simulink model "CM660A_HwTq1Meas"  (R2013b)
settings: Solver=FixedStepDiscrete  StartTime=0.0  StopTime=20  FixedStep=0.002  RelTol=1e-3
undefined symbols (not defined in the file): ELECGLBPRM_HWTQOFFS_HWNWTMTR_F32, ELECGLBPRM_HWTQSATNLOWRLIM_HWNWTMTR_F32, ELECGLBPRM_HWTQSATNUPPRLIM_HWNWTMTR_F32, ELECGLBPRM_HWTQSCA_ULS_F32, ELECGLBPRM_NOFLT_CNT_U08, ELECGLBPRM_OFFSTRIMNOTPRFM_CNT_U08, ELECGLBPRM_PRTCLFLT_CNT_U08, ELECGLBPRM_SNSRINTFLT_CNT_U08, HwTq1MeasHwTq1PrtclFltFailStep, HwTq1MeasHwTq1PrtclFltPassStep, NtcNr1, NtcSts1, RACKLIMRCCWEOTSCA_ULS_F32, RACKLIMRCWEOTSCA_ULS_F32, sigbuilder_block, SigQlfr1
libraries: simulink x25, NxtrNvM x3, NxtrLim x2
(part 2 of 3)

== system CM660A_HwTq1Meas/HwTq1Meas/HwTq1MeasInit1/GetRefTmr1MicroSec32bit ==
  CopyRight2 : Subsystem  Description=|  mask(Copyright Information){none=on}
      | Copyright info block.                                               
      |                                                                     
      | Place copyright information at the top of every subsystem in design.
      mask prompts: none "No parameters"
      mask help: Place copyright information at the top of every subsystem in design.
      mask Display:
      | NxtrConf = 'Nexteer Confidential';
      | 
      | sys = bdroot; %handle for the current model ("system")
      | first = get_param(sys,'Created');
      | first = first(end-3:end);  %year is last four digits
      | 
      | last = get_param(sys,'LastModifiedDate');
      | if isempty(last)
      |     last = datestr(now,'yyyy');
      | else
      |     last = last(end-3:end);
      | end
      | 
      | if strcmp(first,last)
      |     fprintf('%s -- Copyright %s Nexteer',NxtrConf,first)
      | else
      |     fprintf('%s -- %s%s- %s Nexteer',NxtrConf,char(169),first,last)
      | end
  Ground : Ground
  RefTmr : Outport
  wires:
  Ground/1 -> RefTmr/1

== system CM660A_HwTq1Meas/HwTq1Meas/HwTq1MeasInit1/GetTiSpan1MicroSec32bit ==
  RefTmr : Inport
  CopyRight2 : Subsystem  Description=|  mask(Copyright Information){none=on}
      | Copyright info block.                                               
      |                                                                     
      | Place copyright information at the top of every subsystem in design.
      mask prompts: none "No parameters"
      mask help: Place copyright information at the top of every subsystem in design.
      mask Display:
      | NxtrConf = 'Nexteer Confidential';
      | 
      | sys = bdroot; %handle for the current model ("system")
      | first = get_param(sys,'Created');
      | first = first(end-3:end);  %year is last four digits
      | 
      | last = get_param(sys,'LastModifiedDate');
      | if isempty(last)
      |     last = datestr(now,'yyyy');
      | else
      |     last = last(end-3:end);
      | end
      | 
      | if strcmp(first,last)
      |     fprintf('%s -- Copyright %s Nexteer',NxtrConf,first)
      | else
      |     fprintf('%s -- %s%s- %s Nexteer',NxtrConf,char(169),first,last)
      | end
  Ground : Ground
  Terminator : Terminator
  TiSpan : Outport
  wires:
  Ground/1 -> TiSpan/1
  RefTmr/1 -> Terminator/1

== system CM660A_HwTq1Meas/HwTq1Meas/HwTq1MeasInit1/IoHwAb_SetFctPrphlHwTq1 ==
  CopyRight2 : Subsystem  Description=|  mask(Copyright Information){none=on}
      | Copyright info block.                                               
      |                                                                     
      | Place copyright information at the top of every subsystem in design.
      mask prompts: none "No parameters"
      mask help: Place copyright information at the top of every subsystem in design.
      mask Display:
      | NxtrConf = 'Nexteer Confidential';
      | 
      | sys = bdroot; %handle for the current model ("system")
      | first = get_param(sys,'Created');
      | first = first(end-3:end);  %year is last four digits
      | 
      | last = get_param(sys,'LastModifiedDate');
      | if isempty(last)
      |     last = datestr(now,'yyyy');
      | else
      |     last = last(end-3:end);
      | end
      | 
      | if strcmp(first,last)
      |     fprintf('%s -- Copyright %s Nexteer',NxtrConf,first)
      | else
      |     fprintf('%s -- %s%s- %s Nexteer',NxtrConf,char(169),first,last)
      | end

== system CM660A_HwTq1Meas/HwTq1Meas/HwTq1MeasPer1/CopyRight2 ==

== system CM660A_HwTq1Meas/HwTq1Meas/HwTq1MeasPer1/DebStepSelection ==
  TestOk : Inport
  CopyRight2 : Subsystem  Description=|  mask(Copyright Information){none=on}
      | Copyright info block.                                               
      |                                                                     
      | Place copyright information at the top of every subsystem in design.
      mask prompts: none "No parameters"
      mask help: Place copyright information at the top of every subsystem in design.
      mask Display:
      | NxtrConf = 'Nexteer Confidential';
      | 
      | sys = bdroot; %handle for the current model ("system")
      | first = get_param(sys,'Created');
      | first = first(end-3:end);  %year is last four digits
      | 
      | last = get_param(sys,'LastModifiedDate');
      | if isempty(last)
      |     last = datestr(now,'yyyy');
      | else
      |     last = last(end-3:end);
      | end
      | 
      | if strcmp(first,last)
      |     fprintf('%s -- Copyright %s Nexteer',NxtrConf,first)
      | else
      |     fprintf('%s -- %s%s- %s Nexteer',NxtrConf,char(169),first,last)
      | end
  NTCFailStepCal : Constant  Value=HwTq1MeasHwTq1PrtclFltFailStep  VectorParams1D=off
  NTCPassStepCal : Constant  Value=HwTq1MeasHwTq1PrtclFltPassStep
  Switch : Switch  Criteria=u2 > Threshold  Threshold=2
  DebStep : Outport
  wires:
  TestOk/1 -> Switch/2
  NTCPassStepCal/1 -> Switch/3
  Switch/1 -> DebStep/1
  NTCFailStepCal/1 -> Switch/1

== system CM660A_HwTq1Meas/HwTq1Meas/HwTq1MeasPer1/Do nothing ==
  Action Port : ActionPort
  CopyRight2 : Subsystem  Description=|  mask(Copyright Information){none=on}
      | Copyright info block.                                               
      |                                                                     
      | Place copyright information at the top of every subsystem in design.
      mask prompts: none "No parameters"
      mask help: Place copyright information at the top of every subsystem in design.
      mask Display:
      | NxtrConf = 'Nexteer Confidential';
      | 
      | sys = bdroot; %handle for the current model ("system")
      | first = get_param(sys,'Created');
      | first = first(end-3:end);  %year is last four digits
      | 
      | last = get_param(sys,'LastModifiedDate');
      | if isempty(last)
      |     last = datestr(now,'yyyy');
      | else
      |     last = last(end-3:end);
      | end
      | 
      | if strcmp(first,last)
      |     fprintf('%s -- Copyright %s Nexteer',NxtrConf,first)
      | else
      |     fprintf('%s -- %s%s- %s Nexteer',NxtrConf,char(169),first,last)
      | end

== system CM660A_HwTq1Meas/HwTq1Meas/HwTq1MeasPer1/GetNtcQlfr ==
  NtcNr : Inport
  CopyRight2 : Subsystem  Description=|  mask(Copyright Information){none=on}
      | Copyright info block.                                               
      |                                                                     
      | Place copyright information at the top of every subsystem in design.
      mask prompts: none "No parameters"
      mask help: Place copyright information at the top of every subsystem in design.
      mask Display:
      | NxtrConf = 'Nexteer Confidential';
      | 
      | sys = bdroot; %handle for the current model ("system")
      | first = get_param(sys,'Created');
      | first = first(end-3:end);  %year is last four digits
      | 
      | last = get_param(sys,'LastModifiedDate');
      | if isempty(last)
      |     last = datestr(now,'yyyy');
      | else
      |     last = last(end-3:end);
      | end
      | 
      | if strcmp(first,last)
      |     fprintf('%s -- Copyright %s Nexteer',NxtrConf,first)
      | else
      |     fprintf('%s -- %s%s- %s Nexteer',NxtrConf,char(169),first,last)
      | end
  Data Store Read : DataStoreRead  DataStoreName=Ntc0x075Qlfr
  Terminator : Terminator
  NtcQlfr : Outport
  wires:
  NtcNr/1 -> Terminator/1
  Data Store Read/1 -> NtcQlfr/1

== system CM660A_HwTq1Meas/HwTq1Meas/HwTq1MeasPer1/GetNtcQlfr1 ==
  NtcNr : Inport
  CopyRight2 : Subsystem  Description=|  mask(Copyright Information){none=on}
      | Copyright info block.                                               
      |                                                                     
      | Place copyright information at the top of every subsystem in design.
      mask prompts: none "No parameters"
      mask help: Place copyright information at the top of every subsystem in design.
      mask Display:
      | NxtrConf = 'Nexteer Confidential';
      | 
      | sys = bdroot; %handle for the current model ("system")
      | first = get_param(sys,'Created');
      | first = first(end-3:end);  %year is last four digits
      | 
      | last = get_param(sys,'LastModifiedDate');
      | if isempty(last)
      |     last = datestr(now,'yyyy');
      | else
      |     last = last(end-3:end);
      | end
      | 
      | if strcmp(first,last)
      |     fprintf('%s -- Copyright %s Nexteer',NxtrConf,first)
      | else
      |     fprintf('%s -- %s%s- %s Nexteer',NxtrConf,char(169),first,last)
      | end
  Data Store Read : DataStoreRead  DataStoreName=Ntc0x1E1Qlfr
  Terminator : Terminator
  NtcQlfr : Outport
  wires:
  NtcNr/1 -> Terminator/1
  Data Store Read/1 -> NtcQlfr/1

== system CM660A_HwTq1Meas/HwTq1Meas/HwTq1MeasPer1/HwTqCalculation ==
  RawHwTq : Inport
  CopyRight2 : Subsystem  Description=|  mask(Copyright Information){none=on}
      | Copyright info block.                                               
      |                                                                     
      | Place copyright information at the top of every subsystem in design.
      mask prompts: none "No parameters"
      mask help: Place copyright information at the top of every subsystem in design.
      mask Display:
      | NxtrConf = 'Nexteer Confidential';
      | 
      | sys = bdroot; %handle for the current model ("system")
      | first = get_param(sys,'Created');
      | first = first(end-3:end);  %year is last four digits
      | 
      | last = get_param(sys,'LastModifiedDate');
      | if isempty(last)
      |     last = datestr(now,'yyyy');
      | else
      |     last = last(end-3:end);
      | end
      | 
      | if strcmp(first,last)
      |     fprintf('%s -- Copyright %s Nexteer',NxtrConf,first)
      | else
      |     fprintf('%s -- %s%s- %s Nexteer',NxtrConf,char(169),first,last)
      | end
  Data Type Conversion : DataTypeConversion  OutDataTypeStr=single
  Data Type Conversion1 : DataTypeConversion  OutDataTypeStr=single
  HwTqOffs : Constant  Value=ELECGLBPRM_HWTQOFFS_HWNWTMTR_F32  OutDataTypeStr=single
  HwTqSca : Constant  Value=ELECGLBPRM_HWTQSCA_ULS_F32  OutDataTypeStr=single
  Product : Product
  Scope1 : Scope  NumInputPorts=2
      settings: YMin=-5~-5  YMax=5~5  SaveName=ScopeData2
  Substract : Sum  Inputs=+-
  HwTqData : Outport  OutDataTypeStr=single
  wires:
  HwTqSca/1 -> Product/2
  Product/1 -> Data Type Conversion1/1
  HwTqOffs/1 -> Substract/2
  Substract/1 -> Data Type Conversion/1
  RawHwTq/1 -> Product/1, Scope1/1
  Data Type Conversion1/1 -> Substract/1
  Data Type Conversion/1 -> Scope1/2, HwTqData/1

== system CM660A_HwTq1Meas/HwTq1Meas/HwTq1MeasPer1/If Action Subsystem1 ==
  Action Port : ActionPort  ActionType=then
  CopyRight2 : Subsystem  Description=|  mask(Copyright Information){none=on}
      | Copyright info block.                                               
      |                                                                     
      | Place copyright information at the top of every subsystem in design.
      mask prompts: none "No parameters"
      mask help: Place copyright information at the top of every subsystem in design.
      mask Display:
      | NxtrConf = 'Nexteer Confidential';
      | 
      | sys = bdroot; %handle for the current model ("system")
      | first = get_param(sys,'Created');
      | first = first(end-3:end);  %year is last four digits
      | 
      | last = get_param(sys,'LastModifiedDate');
      | if isempty(last)
      |     last = datestr(now,'yyyy');
      | else
      |     last = last(end-3:end);
      | end
      | 
      | if strcmp(first,last)
      |     fprintf('%s -- Copyright %s Nexteer',NxtrConf,first)
      | else
      |     fprintf('%s -- %s%s- %s Nexteer',NxtrConf,char(169),first,last)
      | end
  Data Type Conversion : DataTypeConversion  OutDataTypeStr=uint8
  SigQlfr : simulink/Sources/Enumerated Constant  OutDataTypeStr=Enum: SigQlfr1  Value=SigQlfr1.SIGQLFR_PASSD  SampleTime=inf
  Qlfr : Outport
  wires:
  SigQlfr/1 -> Data Type Conversion/1
  Data Type Conversion/1 -> Qlfr/1

== system CM660A_HwTq1Meas/HwTq1Meas/HwTq1MeasPer1/If Action Subsystem3 ==
  Action Port : ActionPort  ActionType=else
  CopyRight2 : Subsystem  Description=|  mask(Copyright Information){none=on}
      | Copyright info block.                                               
      |                                                                     
      | Place copyright information at the top of every subsystem in design.
      mask prompts: none "No parameters"
      mask help: Place copyright information at the top of every subsystem in design.
      mask Display:
      | NxtrConf = 'Nexteer Confidential';
      | 
      | sys = bdroot; %handle for the current model ("system")
      | first = get_param(sys,'Created');
      | first = first(end-3:end);  %year is last four digits
      | 
      | last = get_param(sys,'LastModifiedDate');
      | if isempty(last)
      |     last = datestr(now,'yyyy');
      | else
      |     last = last(end-3:end);
      | end
      | 
      | if strcmp(first,last)
      |     fprintf('%s -- Copyright %s Nexteer',NxtrConf,first)
      | else
      |     fprintf('%s -- %s%s- %s Nexteer',NxtrConf,char(169),first,last)
      | end
  Data Type Conversion : DataTypeConversion  OutDataTypeStr=uint8
  SigQlfr : simulink/Sources/Enumerated Constant  OutDataTypeStr=Enum: SigQlfr1  Value=SigQlfr1.SIGQLFR_FAILD  SampleTime=inf
  Qlfr : Outport
  wires:
  SigQlfr/1 -> Data Type Conversion/1
  Data Type Conversion/1 -> Qlfr/1

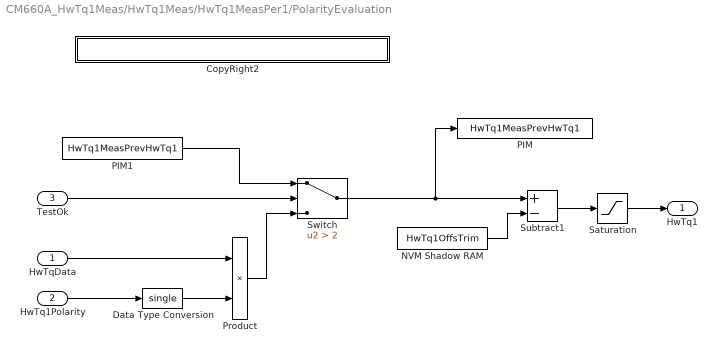
== system CM660A_HwTq1Meas/HwTq1Meas/HwTq1MeasPer1/PolarityEvaluation ==
  HwTqData : Inport  OutDataTypeStr=single
  HwTq1Polarity : Inport  RequirementInfo={} %GIDa_5e7beb6a_cd04_4438_bb0a_c4f4e2c14332  Port=2
  TestOk : Inport  Port=3
  CopyRight2 : Subsystem  Description=|  mask(Copyright Information){none=on}
      | Copyright info block.                                               
      |                                                                     
      | Place copyright information at the top of every subsystem in design.
      mask prompts: none "No parameters"
      mask help: Place copyright information at the top of every subsystem in design.
      mask Display:
      | NxtrConf = 'Nexteer Confidential';
      | 
      | sys = bdroot; %handle for the current model ("system")
      | first = get_param(sys,'Created');
      | first = first(end-3:end);  %year is last four digits
      | 
      | last = get_param(sys,'LastModifiedDate');
      | if isempty(last)
      |     last = datestr(now,'yyyy');
      | else
      |     last = last(end-3:end);
      | end
      | 
      | if strcmp(first,last)
      |     fprintf('%s -- Copyright %s Nexteer',NxtrConf,first)
      | else
      |     fprintf('%s -- %s%s- %s Nexteer',NxtrConf,char(169),first,last)
      | end
  Data Type Conversion : DataTypeConversion  OutDataTypeStr=single
  NVM Shadow RAM : DataStoreRead  DataStoreName=HwTq1OffsTrim
  PIM : DataStoreWrite  RequirementInfo={'doors' '00006115' '14' 'false' 'DOORS Surrogate Item' '' ; 'linktype_rmi_doors' '0000c47c (/ESG Group/FDD Module Requirements/EA4 Specific/CM660A_HwTq1Meas)' '#CM660A_50' 'true' 'REQ: CM660A_50' '' } %GIDa_077e43ec_662e_4d42_809b_03b059cade12  DataStoreName=HwTq1MeasPrevHwTq1
  PIM1 : DataStoreRead  DataStoreName=HwTq1MeasPrevHwTq1
  Product : Product  RequirementInfo={} %GIDa_582e6352_5967_4634_8e9a_a4093cfb2cb3
  Saturation : Saturate  UpperLimit=ELECGLBPRM_HWTQSATNUPPRLIM_HWNWTMTR_F32  LowerLimit=ELECGLBPRM_HWTQSATNLOWRLIM_HWNWTMTR_F32
  Subtract1 : Sum  Inputs=+-
  Switch : Switch  Criteria=u2 > Threshold  Threshold=2
  HwTq1 : Outport  RequirementInfo={'doors' '00006115' '15' 'false' 'DOORS Surrogate Item' '' ; 'linktype_rmi_doors' '0000c47c (/ESG Group/FDD Module Requirements/EA4 Specific/CM660A_HwTq1Meas)' '#CM660A_26' 'true' 'REQ: CM660A_26' '' } %GIDa_69c0e8a1_8bbe_4d59_a878_293d2bf0a501
  wires:
  Product/1 -> Switch/3
  TestOk/1 -> Switch/2
  Switch/1 -> PIM/1, Subtract1/1
  HwTq1Polarity/1 -> Data Type Conversion/1
  HwTqData/1 -> Product/1
  Data Type Conversion/1 -> Product/2
  Saturation/1 -> HwTq1/1
  Subtract1/1 -> Saturation/1
  NVM Shadow RAM/1 -> Subtract1/2
  PIM1/1 -> Switch/1

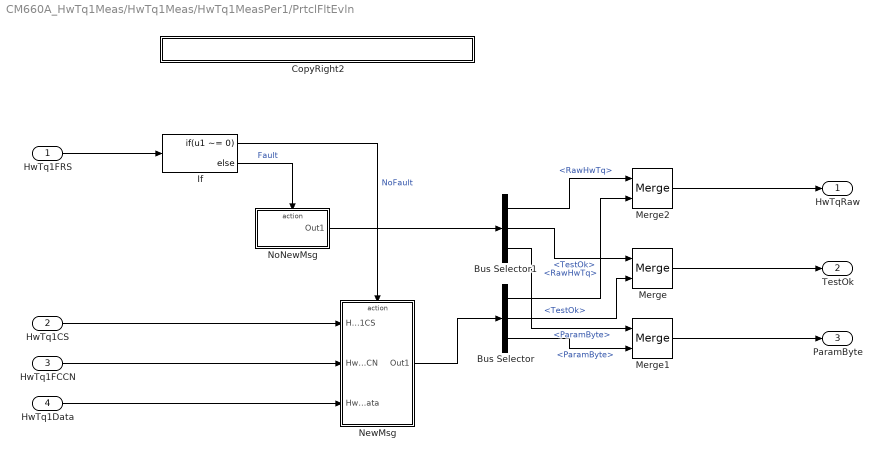
== system CM660A_HwTq1Meas/HwTq1Meas/HwTq1MeasPer1/PrtclFltEvln ==
  HwTq1FRS : Inport
  HwTq1CS : Inport  Port=2
  HwTq1FCCN : Inport  Port=3
  HwTq1Data : Inport  Port=4
  Bus Selector : BusSelector  OutputSignals=RawHwTq,TestOk,ParamByte
  Bus Selector1 : BusSelector  OutputSignals=RawHwTq,TestOk,ParamByte
  CopyRight2 : Subsystem  Description=|  mask(Copyright Information){none=on}
      | Copyright info block.                                               
      |                                                                     
      | Place copyright information at the top of every subsystem in design.
      mask prompts: none "No parameters"
      mask help: Place copyright information at the top of every subsystem in design.
      mask Display:
      | NxtrConf = 'Nexteer Confidential';
      | 
      | sys = bdroot; %handle for the current model ("system")
      | first = get_param(sys,'Created');
      | first = first(end-3:end);  %year is last four digits
      | 
      | last = get_param(sys,'LastModifiedDate');
      | if isempty(last)
      |     last = datestr(now,'yyyy');
      | else
      |     last = last(end-3:end);
      | end
      | 
      | if strcmp(first,last)
      |     fprintf('%s -- Copyright %s Nexteer',NxtrConf,first)
      | else
      |     fprintf('%s -- %s%s- %s Nexteer',NxtrConf,char(169),first,last)
      | end
  If : If  RequirementInfo={} %GIDa_27eddd86_3d73_4bbd_afc6_65cd0e917778  IfExpression=u1 ~= 0
  Merge : Merge
  Merge1 : Merge
  Merge2 : Merge
  NewMsg : Subsystem  RequirementInfo={'doors' '00006115' '17' 'false' 'DOORS Surrogate Item' '' } %GIDa_f428d820_7294_4433_be58_b2aad0418e6b  TreatAsAtomicUnit=on
      mask Display: disp('NewMsg')
  NoNewMsg : Subsystem  RequirementInfo={'doors' '00006115' '22' 'false' 'DOORS Surrogate Item' '' ; 'linktype_rmi_doors' '0000c47c (/ESG Group/FDD Module Requirements/EA4 Specific/CM660A_HwTq1Meas)' '#CM660A_47' 'true' 'REQ: CM660A_47' '' } %GIDa_9ee32e8d_1fd5_4b70_809d_63728be7576b  TreatAsAtomicUnit=on
      mask Display: disp('NoNewMsg')
  HwTqRaw : Outport
  TestOk : Outport  RequirementInfo={} %GIDa_95c6eb83_6b78_451b_a98a_b39fb65983b6  Port=2
  ParamByte : Outport  Port=3
  wires:
  HwTq1FRS/1 -> If/1
  If/1 -> NewMsg/Action  "NoFault"
  If/2 -> NoNewMsg/Action  "Fault"
  HwTq1CS/1 -> NewMsg/1(HwTq1CS)
  Merge/1 -> TestOk/1
  Merge1/1 -> ParamByte/1
  Merge2/1 -> HwTqRaw/1
  NewMsg/1(Out1) -> Bus Selector/1
  NoNewMsg/1(Out1) -> Bus Selector1/1
  Bus Selector1/1 -> Merge2/1  "<RawHwTq>"
  Bus Selector/1 -> Merge2/2  "<RawHwTq>"
  Bus Selector1/2 -> Merge/1  "<TestOk>"
  Bus Selector1/3 -> Merge1/1  "<ParamByte>"
  Bus Selector/2 -> Merge/2  "<TestOk>"
  Bus Selector/3 -> Merge1/2  "<ParamByte>"
  HwTq1FCCN/1 -> NewMsg/2(HwTq1FCCN)
  HwTq1Data/1 -> NewMsg/3(HwTq1Data)

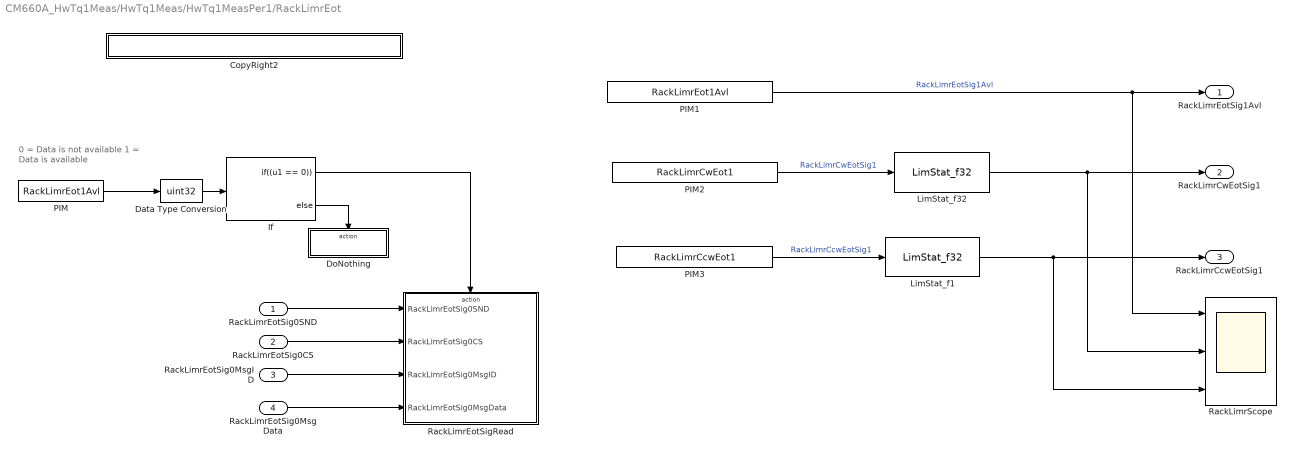
== system CM660A_HwTq1Meas/HwTq1Meas/HwTq1MeasPer1/RackLimrEot ==
  note: 0 = Data is not available
      | 1 = Data is available
  RackLimrEotSig0SND : Inport
  RackLimrEotSig0CS : Inport  Port=2
  RackLimrEotSig0MsgID : Inport  Port=3
  RackLimrEotSig0MsgData : Inport  Port=4
  CopyRight2 : Subsystem  Description=|  mask(Copyright Information){none=on}
      | Copyright info block.                                               
      |                                                                     
      | Place copyright information at the top of every subsystem in design.
      mask prompts: none "No parameters"
      mask help: Place copyright information at the top of every subsystem in design.
      mask Display:
      | NxtrConf = 'Nexteer Confidential';
      | 
      | sys = bdroot; %handle for the current model ("system")
      | first = get_param(sys,'Created');
      | first = first(end-3:end);  %year is last four digits
      | 
      | last = get_param(sys,'LastModifiedDate');
      | if isempty(last)
      |     last = datestr(now,'yyyy');
      | else
      |     last = last(end-3:end);
      | end
      | 
      | if strcmp(first,last)
      |     fprintf('%s -- Copyright %s Nexteer',NxtrConf,first)
      | else
      |     fprintf('%s -- %s%s- %s Nexteer',NxtrConf,char(169),first,last)
      | end
  Data Type Conversion : DataTypeConversion  OutDataTypeStr=uint32
  DoNothing : Subsystem  TreatAsAtomicUnit=on
  If : If  RequirementInfo={'linktype_rmi_doors' '0000c47c (/ESG Group/FDD Module Requirements/EA4 Specific/CM660A_HwTq1Meas)' '#CM660A_76' 'true' 'REQ: CM660A_76' '' } %GIDa_97ae3cdc_ee3b_4209_9f7f_e3776c69d98b  IfExpression=(u1 == 0)
  LimStat_f1 : NxtrLim/LimStat_f32  LoLim=RACKLIMREOTSIGLOLIM_HWDEG_F32  HiLim=0
      settings: AttributesFormatString=|
      | Low Limit: %<LoLim>
      | High Limit:%<HiLim>
  LimStat_f32 : NxtrLim/LimStat_f32  LoLim=0  HiLim=RACKLIMREOTSIGHILIM_HWDEG_F32
      settings: AttributesFormatString=|
      | Low Limit: %<LoLim>
      | High Limit:%<HiLim>
  PIM : DataStoreRead  DataStoreName=RackLimrEot1Avl
  PIM1 : DataStoreRead  RequirementInfo={'linktype_rmi_doors' '0000c47c (/ESG Group/FDD Module Requirements/EA4 Specific/CM660A_HwTq1Meas)' '#CM660A_75' 'true' 'REQ: CM660A_75' '' } %GIDa_392854b3_63b2_4906_80b7_a431b4afe123  DataStoreName=RackLimrEot1Avl
  PIM2 : DataStoreRead  RequirementInfo={'linktype_rmi_doors' '0000c47c (/ESG Group/FDD Module Requirements/EA4 Specific/CM660A_HwTq1Meas)' '#CM660A_70' 'true' 'REQ: CM660A_70' '' } %GIDa_17573b11_b989_4fbe_97c8_53900f7d59bd  DataStoreName=RackLimrCwEot1
  PIM3 : DataStoreRead  RequirementInfo={'linktype_rmi_doors' '0000c47c (/ESG Group/FDD Module Requirements/EA4 Specific/CM660A_HwTq1Meas)' '#CM660A_70' 'true' 'REQ: CM660A_70' '' } %GIDa_738d479f_26d5_4ed1_ad08_c0c77187e1ac  DataStoreName=RackLimrCcwEot1
  RackLimrEotSigRead : Subsystem  TreatAsAtomicUnit=on
  RackLimrScope : Scope  NumInputPorts=3
      settings: ShowLegends=on  TimeRange=20  YMin=-1~-100~-600  YMax=2~700~100
  RackLimrEotSig1Avl : Outport  RequirementInfo={} %GIDa_e207e200_0be5_4dbd_b5aa_9dcd133582ed
  RackLimrCwEotSig1 : Outport  RequirementInfo={} %GIDa_d68e745f_bbf7_4a55_9745_7febacfcaae5  Port=2
  RackLimrCcwEotSig1 : Outport  RequirementInfo={} %GIDa_d2e09d57_2587_426a_a7f5_ae8ec9b64963  Port=3
  wires:
  PIM/1 -> Data Type Conversion/1
  Data Type Conversion/1 -> If/1
  If/2 -> DoNothing/Action
  If/1 -> RackLimrEotSigRead/Action
  PIM2/1 -> LimStat_f32/1  "RackLimrCwEotSig1"
  PIM3/1 -> LimStat_f1/1  "RackLimrCcwEotSig1"
  PIM1/1 -> RackLimrScope/1, RackLimrEotSig1Avl/1  "RackLimrEotSig1Avl"
  LimStat_f32/1 -> RackLimrScope/2, RackLimrCwEotSig1/1
  LimStat_f1/1 -> RackLimrScope/3, RackLimrCcwEotSig1/1
  RackLimrEotSig0SND/1 -> RackLimrEotSigRead/1(RackLimrEotSig0SND)
  RackLimrEotSig0MsgID/1 -> RackLimrEotSigRead/3(RackLimrEotSig0MsgID)
  RackLimrEotSig0CS/1 -> RackLimrEotSigRead/2(RackLimrEotSig0CS)
  RackLimrEotSig0MsgData/1 -> RackLimrEotSigRead/4(RackLimrEotSig0MsgData)

== system CM660A_HwTq1Meas/HwTq1Meas/HwTq1MeasPer1/Read the Flag ==
  RegInpRSENT1FND : Inport
  Action Port : ActionPort
  CopyRight2 : Subsystem  Description=|  mask(Copyright Information){none=on}
      | Copyright info block.                                               
      |                                                                     
      | Place copyright information at the top of every subsystem in design.
      mask prompts: none "No parameters"
      mask help: Place copyright information at the top of every subsystem in design.
      mask Display:
      | NxtrConf = 'Nexteer Confidential';
      | 
      | sys = bdroot; %handle for the current model ("system")
      | first = get_param(sys,'Created');
      | first = first(end-3:end);  %year is last four digits
      | 
      | last = get_param(sys,'LastModifiedDate');
      | if isempty(last)
      |     last = datestr(now,'yyyy');
      | else
      |     last = last(end-3:end);
      | end
      | 
      | if strcmp(first,last)
      |     fprintf('%s -- Copyright %s Nexteer',NxtrConf,first)
      | else
      |     fprintf('%s -- %s%s- %s Nexteer',NxtrConf,char(169),first,last)
      | end
  RSENT1DummyRead : Terminator
  wires:
  RegInpRSENT1FND/1 -> RSENT1DummyRead/1

== system CM660A_HwTq1Meas/HwTq1Meas/HwTq1MeasPer1/SetNtcSts ==
  note: Note:
      |
      | - "ISO Fault Debounce Design" Simulink block intent to use here for Simulation purpose only. Do not Code this block
  NtcNr : Inport
  NtcStInfo : Inport  Port=2
  NtcSts : Inport  Port=3
  DebStep : Inport  Port=4
  CopyRight2 : Subsystem  Description=|  mask(Copyright Information){none=on}
      | Copyright info block.                                               
      |                                                                     
      | Place copyright information at the top of every subsystem in design.
      mask prompts: none "No parameters"
      mask help: Place copyright information at the top of every subsystem in design.
      mask Display:
      | NxtrConf = 'Nexteer Confidential';
      | 
      | sys = bdroot; %handle for the current model ("system")
      | first = get_param(sys,'Created');
      | first = first(end-3:end);  %year is last four digits
      | 
      | last = get_param(sys,'LastModifiedDate');
      | if isempty(last)
      |     last = datestr(now,'yyyy');
      | else
      |     last = last(end-3:end);
      | end
      | 
      | if strcmp(first,last)
      |     fprintf('%s -- Copyright %s Nexteer',NxtrConf,first)
      | else
      |     fprintf('%s -- %s%s- %s Nexteer',NxtrConf,char(169),first,last)
      | end
  Data Store Write : DataStoreWrite  DataStoreName=Ntc0x075Qlfr
  Ground : Ground
  ISO Fault Debounce Design : Stateflow chart  TreatAsAtomicUnit=on
      settings: AttributesFormatString=|
      | Simulation Purpose Only.
      | Do Not Code this block
      | Diagnostic Manager Owns this requirement
  Scope1 : Scope  NumInputPorts=3
      settings: YMin=-5~-5~-5  YMax=5~5~5  SaveName=ScopeData5
  Terminator : Terminator
  Terminator1 : Terminator
  wires:
  NtcStInfo/1 -> Terminator1/1
  NtcNr/1 -> Terminator/1
  NtcSts/1 -> ISO Fault Debounce Design/1(NtcSts), Scope1/1
  DebStep/1 -> ISO Fault Debounce Design/2(DebStep), Scope1/2
  ISO Fault Debounce Design/1(Qualifier) -> Scope1/3, Data Store Write/1
  Ground/1 -> ISO Fault Debounce Design/3(SvcClr)

== system CM660A_HwTq1Meas/HwTq1Meas/HwTq1MeasPer2/CopyRight2 ==

== system CM660A_HwTq1Meas/HwTq1Meas/HwTq1MeasPer2/If Action Subsystem ==
  Action Port : ActionPort  ActionType=then
  CopyRight2 : Subsystem  Description=|  mask(Copyright Information){none=on}
      | Copyright info block.                                               
      |                                                                     
      | Place copyright information at the top of every subsystem in design.
      mask prompts: none "No parameters"
      mask help: Place copyright information at the top of every subsystem in design.
      mask Display:
      | NxtrConf = 'Nexteer Confidential';
      | 
      | sys = bdroot; %handle for the current model ("system")
      | first = get_param(sys,'Created');
      | first = first(end-3:end);  %year is last four digits
      | 
      | last = get_param(sys,'LastModifiedDate');
      | if isempty(last)
      |     last = datestr(now,'yyyy');
      | else
      |     last = last(end-3:end);
      | end
      | 
      | if strcmp(first,last)
      |     fprintf('%s -- Copyright %s Nexteer',NxtrConf,first)
      | else
      |     fprintf('%s -- %s%s- %s Nexteer',NxtrConf,char(169),first,last)
      | end
  Data Type Conversion : DataTypeConversion  OutDataTypeStr=uint8
  NoFlt : Constant  RequirementInfo={} %GIDa_73f0a11e_cf31_48e6_8bb2_3cf4b1949e36  Value=ELECGLBPRM_NOFLT_CNT_U08  OutDataTypeStr=uint8
  NtcSts : simulink/Sources/Enumerated Constant  OutDataTypeStr=Enum: NtcSts1  Value=NtcSts1.NTCSTS_PASSD  SampleTime=inf
  ParamByte : Outport
  TestOk : Outport  Port=2
  wires:
  NtcSts/1 -> Data Type Conversion/1
  NoFlt/1 -> ParamByte/1
  Data Type Conversion/1 -> TestOk/1

== system CM660A_HwTq1Meas/HwTq1Meas/HwTq1MeasPer2/If Action Subsystem1 ==
  Action Port : ActionPort  ActionType=else
  CopyRight2 : Subsystem  Description=|  mask(Copyright Information){none=on}
      | Copyright info block.                                               
      |                                                                     
      | Place copyright information at the top of every subsystem in design.
      mask prompts: none "No parameters"
      mask help: Place copyright information at the top of every subsystem in design.
      mask Display:
      | NxtrConf = 'Nexteer Confidential';
      | 
      | sys = bdroot; %handle for the current model ("system")
      | first = get_param(sys,'Created');
      | first = first(end-3:end);  %year is last four digits
      | 
      | last = get_param(sys,'LastModifiedDate');
      | if isempty(last)
      |     last = datestr(now,'yyyy');
      | else
      |     last = last(end-3:end);
      | end
      | 
      | if strcmp(first,last)
      |     fprintf('%s -- Copyright %s Nexteer',NxtrConf,first)
      | else
      |     fprintf('%s -- %s%s- %s Nexteer',NxtrConf,char(169),first,last)
      | end
  Data Type Conversion : DataTypeConversion  OutDataTypeStr=uint8
  NoFlt : Constant  RequirementInfo={} %GIDa_eae82ea4_69e1_4b6f_94ef_18d1f1394a46  Value=ELECGLBPRM_OFFSTRIMNOTPRFM_CNT_U08  OutDataTypeStr=uint8
  NtcSts : simulink/Sources/Enumerated Constant  OutDataTypeStr=Enum: NtcSts1  Value=NtcSts1.NTCSTS_FAILD  SampleTime=inf
  ParamByte : Outport
  TestOk : Outport  Port=2
  wires:
  NoFlt/1 -> ParamByte/1
  NtcSts/1 -> Data Type Conversion/1
  Data Type Conversion/1 -> TestOk/1

== system CM660A_HwTq1Meas/HwTq1Meas/HwTq1MeasPer2/SetNtcSts ==
  note: Note:
      |
      | - "ISO Fault Debounce Design" Simulink block intent to use here for Simulation purpose only. Do not Code this block
  NtcNr : Inport
  NtcStInfo : Inport  Port=2
  NtcSts : Inport  Port=3
  DebStep : Inport  Port=4
  CopyRight2 : Subsystem  Description=|  mask(Copyright Information){none=on}
      | Copyright info block.                                               
      |                                                                     
      | Place copyright information at the top of every subsystem in design.
      mask prompts: none "No parameters"
      mask help: Place copyright information at the top of every subsystem in design.
      mask Display:
      | NxtrConf = 'Nexteer Confidential';
      | 
      | sys = bdroot; %handle for the current model ("system")
      | first = get_param(sys,'Created');
      | first = first(end-3:end);  %year is last four digits
      | 
      | last = get_param(sys,'LastModifiedDate');
      | if isempty(last)
      |     last = datestr(now,'yyyy');
      | else
      |     last = last(end-3:end);
      | end
      | 
      | if strcmp(first,last)
      |     fprintf('%s -- Copyright %s Nexteer',NxtrConf,first)
      | else
      |     fprintf('%s -- %s%s- %s Nexteer',NxtrConf,char(169),first,last)
      | end
  Data Store Write : DataStoreWrite  DataStoreName=Ntc0x1E1Qlfr
  Ground : Ground
  ISO Fault Debounce Design : Stateflow chart  TreatAsAtomicUnit=on
      settings: AttributesFormatString=|
      | Simulation Purpose Only.
      | Do Not Code this block
      | Diagnostic Manager Owns this requirement
  Scope1 : Scope  NumInputPorts=3
      settings: YMin=-5~-5~-5  YMax=5~5~5  SaveName=ScopeData5
  Terminator : Terminator
  Terminator1 : Terminator
  wires:
  Ground/1 -> ISO Fault Debounce Design/3(SvcClr)
  ISO Fault Debounce Design/1(Qualifier) -> Data Store Write/1, Scope1/3
  DebStep/1 -> Scope1/2, ISO Fault Debounce Design/2(DebStep)
  NtcSts/1 -> Scope1/1, ISO Fault Debounce Design/1(NtcSts)
  NtcNr/1 -> Terminator/1
  NtcStInfo/1 -> Terminator1/1

== system CM660A_HwTq1Meas/HwTq1Meas/HwTq1MeasTrigStrt/CopyRight2 ==

== system CM660A_HwTq1Meas/HwTq1Meas/HwTq1MeasTrigStrt/GetRefTmr1MicroSec32bit ==
  CopyRight2 : Subsystem  Description=|  mask(Copyright Information){none=on}
      | Copyright info block.                                               
      |                                                                     
      | Place copyright information at the top of every subsystem in design.
      mask prompts: none "No parameters"
      mask help: Place copyright information at the top of every subsystem in design.
      mask Display:
      | NxtrConf = 'Nexteer Confidential';
      | 
      | sys = bdroot; %handle for the current model ("system")
      | first = get_param(sys,'Created');
      | first = first(end-3:end);  %year is last four digits
      | 
      | last = get_param(sys,'LastModifiedDate');
      | if isempty(last)
      |     last = datestr(now,'yyyy');
      | else
      |     last = last(end-3:end);
      | end
      | 
      | if strcmp(first,last)
      |     fprintf('%s -- Copyright %s Nexteer',NxtrConf,first)
      | else
      |     fprintf('%s -- %s%s- %s Nexteer',NxtrConf,char(169),first,last)
      | end
  Ground : Ground
  RefTmr : Outport
  wires:
  Ground/1 -> RefTmr/1

== system CM660A_HwTq1Meas/HwTq1Meas/HwTq1MeasTrigStrt/GetTiSpan1MicroSec32bit ==
  RefTmr : Inport
  CopyRight2 : Subsystem  Description=|  mask(Copyright Information){none=on}
      | Copyright info block.                                               
      |                                                                     
      | Place copyright information at the top of every subsystem in design.
      mask prompts: none "No parameters"
      mask help: Place copyright information at the top of every subsystem in design.
      mask Display:
      | NxtrConf = 'Nexteer Confidential';
      | 
      | sys = bdroot; %handle for the current model ("system")
      | first = get_param(sys,'Created');
      | first = first(end-3:end);  %year is last four digits
      | 
      | last = get_param(sys,'LastModifiedDate');
      | if isempty(last)
      |     last = datestr(now,'yyyy');
      | else
      |     last = last(end-3:end);
      | end
      | 
      | if strcmp(first,last)
      |     fprintf('%s -- Copyright %s Nexteer',NxtrConf,first)
      | else
      |     fprintf('%s -- %s%s- %s Nexteer',NxtrConf,char(169),first,last)
      | end
  Ground : Ground
  Terminator : Terminator
  TiSpan : Outport
  wires:
  RefTmr/1 -> Terminator/1
  Ground/1 -> TiSpan/1

== system CM660A_HwTq1Meas/HwTq1Meas/HwTq1MeasInit1/GetRefTmr1MicroSec32bit/CopyRight2 ==

== system CM660A_HwTq1Meas/HwTq1Meas/HwTq1MeasInit1/GetTiSpan1MicroSec32bit/CopyRight2 ==

== system CM660A_HwTq1Meas/HwTq1Meas/HwTq1MeasInit1/IoHwAb_SetFctPrphlHwTq1/CopyRight2 ==

== system CM660A_HwTq1Meas/HwTq1Meas/HwTq1MeasPer1/DebStepSelection/CopyRight2 ==

== system CM660A_HwTq1Meas/HwTq1Meas/HwTq1MeasPer1/Do nothing/CopyRight2 ==

== system CM660A_HwTq1Meas/HwTq1Meas/HwTq1MeasPer1/GetNtcQlfr/CopyRight2 ==

== system CM660A_HwTq1Meas/HwTq1Meas/HwTq1MeasPer1/GetNtcQlfr1/CopyRight2 ==

== system CM660A_HwTq1Meas/HwTq1Meas/HwTq1MeasPer1/HwTqCalculation/CopyRight2 ==

== system CM660A_HwTq1Meas/HwTq1Meas/HwTq1MeasPer1/If Action Subsystem1/CopyRight2 ==

== system CM660A_HwTq1Meas/HwTq1Meas/HwTq1MeasPer1/If Action Subsystem3/CopyRight2 ==

== system CM660A_HwTq1Meas/HwTq1Meas/HwTq1MeasPer1/PolarityEvaluation/CopyRight2 ==

== system CM660A_HwTq1Meas/HwTq1Meas/HwTq1MeasPer1/PrtclFltEvln/CopyRight2 ==

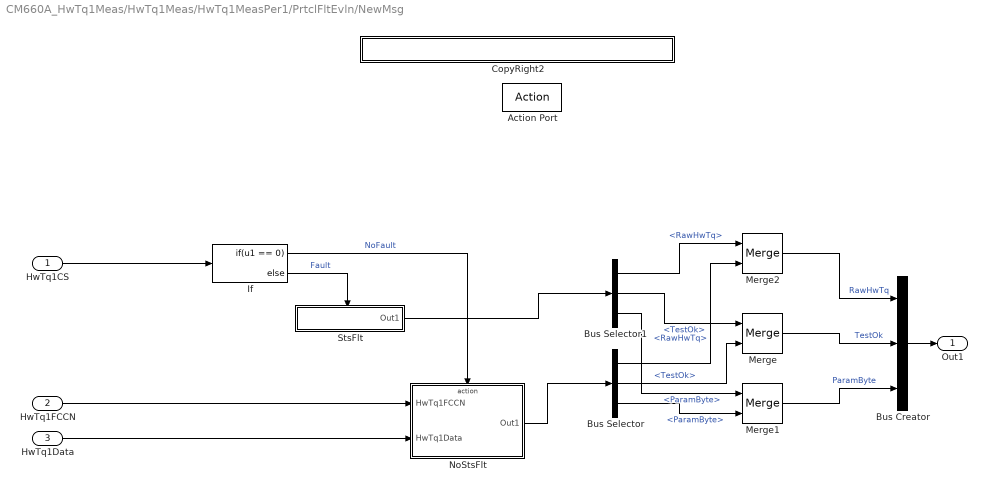
== system CM660A_HwTq1Meas/HwTq1Meas/HwTq1MeasPer1/PrtclFltEvln/NewMsg ==
  HwTq1CS : Inport
  HwTq1FCCN : Inport  Port=2
  HwTq1Data : Inport  Port=3
  Action Port : ActionPort  ActionType=then
  Bus Creator : BusCreator  Inputs=3
  Bus Selector : BusSelector  OutputSignals=RawHwTq,TestOk,ParamByte
  Bus Selector1 : BusSelector  OutputSignals=RawHwTq,TestOk,ParamByte
  CopyRight2 : Subsystem  Description=|  mask(Copyright Information){none=on}
      | Copyright info block.                                               
      |                                                                     
      | Place copyright information at the top of every subsystem in design.
      mask prompts: none "No parameters"
      mask help: Place copyright information at the top of every subsystem in design.
      mask Display:
      | NxtrConf = 'Nexteer Confidential';
      | 
      | sys = bdroot; %handle for the current model ("system")
      | first = get_param(sys,'Created');
      | first = first(end-3:end);  %year is last four digits
      | 
      | last = get_param(sys,'LastModifiedDate');
      | if isempty(last)
      |     last = datestr(now,'yyyy');
      | else
      |     last = last(end-3:end);
      | end
      | 
      | if strcmp(first,last)
      |     fprintf('%s -- Copyright %s Nexteer',NxtrConf,first)
      | else
      |     fprintf('%s -- %s%s- %s Nexteer',NxtrConf,char(169),first,last)
      | end
  If : If  IfExpression=u1 == 0
  Merge : Merge
  Merge1 : Merge
  Merge2 : Merge
  NoStsFlt : Subsystem  RequirementInfo={'doors' '00006115' '18' 'false' 'DOORS Surrogate Item' '' } %GIDa_ac6611b7_c860_4920_977e_a7e9bf2750f4  TreatAsAtomicUnit=on
  StsFlt : Subsystem  RequirementInfo={'doors' '00006115' '21' 'false' 'DOORS Surrogate Item' '' ; 'linktype_rmi_doors' '0000c47c (/ESG Group/FDD Module Requirements/EA4 Specific/CM660A_HwTq1Meas)' '#CM660A_40' 'true' 'REQ: CM660A_40' '' ; 'linktype_rmi_doors' '0000c47c (/ESG Group/FDD Module Requirements/EA4 Specific/CM660A_HwTq1Meas)' '#CM660A_41' 'true' 'REQ: CM660A_41' '' ; 'linktype_rmi_doors' '0000c47c (/ESG Group/FDD Module Requirements/EA4 Specific/CM660A_HwTq1Meas)' '#CM660A_42' 'true' 'REQ: CM660A_42' '' ; 'linktype_rmi_doors' '0000c47c (/ESG Group/FDD Module Requirements/EA4 Specific/CM660A_HwTq1Meas)' '#CM660A_43' 'true' 'REQ: CM660A_43' '' ; 'linktype_rmi_doors' '0000c47c (/ESG Group/FDD Module Requirements/EA4 Specific/CM660A_HwTq1Meas)' '#CM660A_44' 'true' 'REQ: CM660A_44' '' ; 'linktype_rmi_doors' '0000c47c (/ESG Group/FDD Module Requirements/EA4 Specific/CM660A_HwTq1Meas)' '#CM660A_45' 'true' 'REQ: CM660A_45' '' ; 'linktype_rmi_doors' '0000c47c (/ESG Group/FDD Module Requirements/EA4 Specific/CM660A_HwTq1Meas)' '#CM660A_46' 'true' 'REQ: CM660A_46' '' } %GIDa_679ffcb4_3849_4021_9957_65733ff452c6  TreatAsAtomicUnit=on
      mask Display: disp('STSFLT')
  Out1 : Outport
  wires:
  If/1 -> NoStsFlt/Action  "NoFault"
  If/2 -> StsFlt/Action  "Fault"
  Merge/1 -> Bus Creator/2  "TestOk"
  Merge1/1 -> Bus Creator/3  "ParamByte"
  Merge2/1 -> Bus Creator/1  "RawHwTq"
  NoStsFlt/1(Out1) -> Bus Selector/1
  StsFlt/1(Out1) -> Bus Selector1/1
  Bus Selector1/1 -> Merge2/1  "<RawHwTq>"
  Bus Selector/1 -> Merge2/2  "<RawHwTq>"
  Bus Selector1/2 -> Merge/1  "<TestOk>"
  Bus Selector1/3 -> Merge1/1  "<ParamByte>"
  Bus Selector/2 -> Merge/2  "<TestOk>"
  Bus Selector/3 -> Merge1/2  "<ParamByte>"
  Bus Creator/1 -> Out1/1
  HwTq1CS/1 -> If/1
  HwTq1FCCN/1 -> NoStsFlt/1(HwTq1FCCN)
  HwTq1Data/1 -> NoStsFlt/2(HwTq1Data)

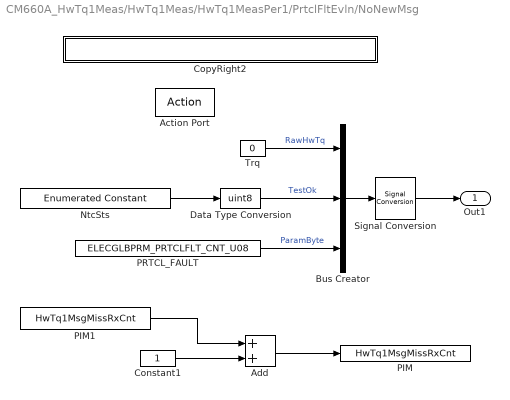
== system CM660A_HwTq1Meas/HwTq1Meas/HwTq1MeasPer1/PrtclFltEvln/NoNewMsg ==
  Action Port : ActionPort  ActionType=else
  Add : Sum
  Bus Creator : BusCreator  Inputs=3
  Constant1 : Constant  OutDataTypeStr=uint32
  CopyRight2 : Subsystem  Description=|  mask(Copyright Information){none=on}
      | Copyright info block.                                               
      |                                                                     
      | Place copyright information at the top of every subsystem in design.
      mask prompts: none "No parameters"
      mask help: Place copyright information at the top of every subsystem in design.
      mask Display:
      | NxtrConf = 'Nexteer Confidential';
      | 
      | sys = bdroot; %handle for the current model ("system")
      | first = get_param(sys,'Created');
      | first = first(end-3:end);  %year is last four digits
      | 
      | last = get_param(sys,'LastModifiedDate');
      | if isempty(last)
      |     last = datestr(now,'yyyy');
      | else
      |     last = last(end-3:end);
      | end
      | 
      | if strcmp(first,last)
      |     fprintf('%s -- Copyright %s Nexteer',NxtrConf,first)
      | else
      |     fprintf('%s -- %s%s- %s Nexteer',NxtrConf,char(169),first,last)
      | end
  Data Type Conversion : DataTypeConversion  OutDataTypeStr=uint8
  NtcSts : simulink/Sources/Enumerated Constant  OutDataTypeStr=Enum: NtcSts1  Value=NtcSts1.NTCSTS_PREFAILD  SampleTime=inf
  PIM : DataStoreWrite  RequirementInfo={} %GIDa_d7aaed20_af5c_45d0_a82c_a669b9da5dc5  DataStoreName=HwTq1MsgMissRxCnt
  PIM1 : DataStoreRead  DataStoreName=HwTq1MsgMissRxCnt
  PRTCL_FAULT : Constant  Value=ELECGLBPRM_PRTCLFLT_CNT_U08  OutDataTypeStr=uint8
  Signal Conversion : SignalConversion
  Trq : Constant  Value=0  OutDataTypeStr=uint32
  Out1 : Outport
  wires:
  NtcSts/1 -> Data Type Conversion/1
  PRTCL_FAULT/1 -> Bus Creator/3  "ParamByte"
  Data Type Conversion/1 -> Bus Creator/2  "TestOk"
  Trq/1 -> Bus Creator/1  "RawHwTq"
  Bus Creator/1 -> Signal Conversion/1
  Signal Conversion/1 -> Out1/1
  Add/1 -> PIM/1
  Constant1/1 -> Add/2
  PIM1/1 -> Add/1

== system CM660A_HwTq1Meas/HwTq1Meas/HwTq1MeasPer1/RackLimrEot/CopyRight2 ==

== system CM660A_HwTq1Meas/HwTq1Meas/HwTq1MeasPer1/RackLimrEot/DoNothing ==
  Action Port : ActionPort  ActionType=else
  CopyRight2 : Subsystem  Description=|  mask(Copyright Information){none=on}
      | Copyright info block.                                               
      |                                                                     
      | Place copyright information at the top of every subsystem in design.
      mask prompts: none "No parameters"
      mask help: Place copyright information at the top of every subsystem in design.
      mask Display:
      | NxtrConf = 'Nexteer Confidential';
      | 
      | sys = bdroot; %handle for the current model ("system")
      | first = get_param(sys,'Created');
      | first = first(end-3:end);  %year is last four digits
      | 
      | last = get_param(sys,'LastModifiedDate');
      | if isempty(last)
      |     last = datestr(now,'yyyy');
      | else
      |     last = last(end-3:end);
      | end
      | 
      | if strcmp(first,last)
      |     fprintf('%s -- Copyright %s Nexteer',NxtrConf,first)
      | else
      |     fprintf('%s -- %s%s- %s Nexteer',NxtrConf,char(169),first,last)
      | end

== system CM660A_HwTq1Meas/HwTq1Meas/HwTq1MeasPer1/RackLimrEot/RackLimrEotSigRead ==
  RackLimrEotSig0SND : Inport
  RackLimrEotSig0CS : Inport  Port=2
  RackLimrEotSig0MsgID : Inport  Port=3
  RackLimrEotSig0MsgData : Inport  Port=4
  Action Port : ActionPort  ActionType=then
  CopyRight2 : Subsystem  Description=|  mask(Copyright Information){none=on}
      | Copyright info block.                                               
      |                                                                     
      | Place copyright information at the top of every subsystem in design.
      mask prompts: none "No parameters"
      mask help: Place copyright information at the top of every subsystem in design.
      mask Display:
      | NxtrConf = 'Nexteer Confidential';
      | 
      | sys = bdroot; %handle for the current model ("system")
      | first = get_param(sys,'Created');
      | first = first(end-3:end);  %year is last four digits
      | 
      | last = get_param(sys,'LastModifiedDate');
      | if isempty(last)
      |     last = datestr(now,'yyyy');
      | else
      |     last = last(end-3:end);
      | end
      | 
      | if strcmp(first,last)
      |     fprintf('%s -- Copyright %s Nexteer',NxtrConf,first)
      | else
      |     fprintf('%s -- %s%s- %s Nexteer',NxtrConf,char(169),first,last)
      | end
  DoNothing1 : Subsystem  TreatAsAtomicUnit=on
  If2 : If  NumInputs=2  IfExpression=(u1 ~= 0)&(u2==0)
  RackLimrEotSigRead1 : Subsystem  RequirementInfo={} %GIDa_34300204_2498_4445_ae4d_7fb71a7a48c5  TreatAsAtomicUnit=on
  wires:
  If2/1 -> RackLimrEotSigRead1/Action
  If2/2 -> DoNothing1/Action
  RackLimrEotSig0SND/1 -> If2/1
  RackLimrEotSig0CS/1 -> If2/2
  RackLimrEotSig0MsgID/1 -> RackLimrEotSigRead1/1(RackLimrEotSig0MsgID)
  RackLimrEotSig0MsgData/1 -> RackLimrEotSigRead1/2(RackLimrEotSig0MsgData)

== system CM660A_HwTq1Meas/HwTq1Meas/HwTq1MeasPer1/Read the Flag/CopyRight2 ==

== system CM660A_HwTq1Meas/HwTq1Meas/HwTq1MeasPer1/SetNtcSts/CopyRight2 ==

== system CM660A_HwTq1Meas/HwTq1Meas/HwTq1MeasPer2/If Action Subsystem/CopyRight2 ==

== system CM660A_HwTq1Meas/HwTq1Meas/HwTq1MeasPer2/If Action Subsystem1/CopyRight2 ==

== system CM660A_HwTq1Meas/HwTq1Meas/HwTq1MeasPer2/SetNtcSts/CopyRight2 ==

== system CM660A_HwTq1Meas/HwTq1Meas/HwTq1MeasTrigStrt/GetRefTmr1MicroSec32bit/CopyRight2 ==

== system CM660A_HwTq1Meas/HwTq1Meas/HwTq1MeasTrigStrt/GetTiSpan1MicroSec32bit/CopyRight2 ==

== system CM660A_HwTq1Meas/HwTq1Meas/HwTq1MeasPer1/PrtclFltEvln/NewMsg/CopyRight2 ==

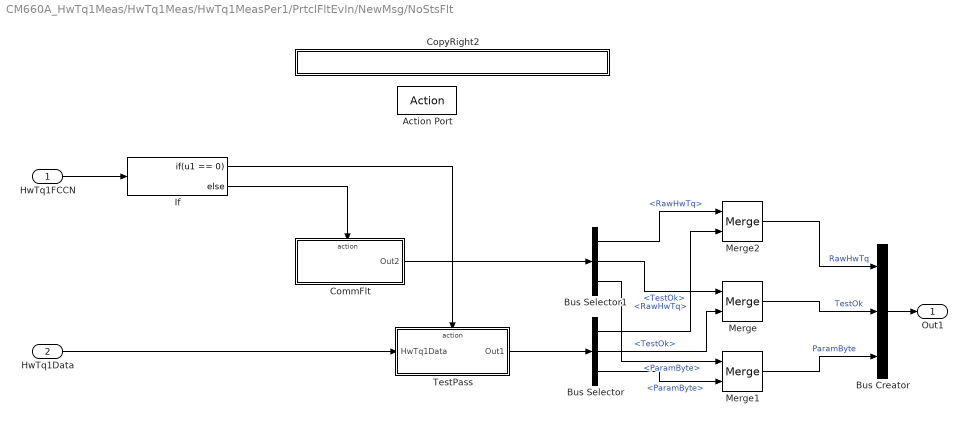
== system CM660A_HwTq1Meas/HwTq1Meas/HwTq1MeasPer1/PrtclFltEvln/NewMsg/NoStsFlt ==
  HwTq1FCCN : Inport
  HwTq1Data : Inport  Port=2
  Action Port : ActionPort  ActionType=then
  Bus Creator : BusCreator  Inputs=3
  Bus Selector : BusSelector  OutputSignals=RawHwTq,TestOk,ParamByte
  Bus Selector1 : BusSelector  OutputSignals=RawHwTq,TestOk,ParamByte
  CommFlt : Subsystem  RequirementInfo={'doors' '00006115' '19' 'false' 'DOORS Surrogate Item' '' ; 'linktype_rmi_doors' '0000c47c (/ESG Group/FDD Module Requirements/EA4 Specific/CM660A_HwTq1Meas)' '#CM660A_28' 'true' 'REQ: CM660A_28' '' ; 'linktype_rmi_doors' '0000c47c (/ESG Group/FDD Module Requirements/EA4 Specific/CM660A_HwTq1Meas)' '#CM660A_48' 'true' 'REQ: CM660A_48' '' } %GIDa_a181911d_9433_49e5_ad17_4bc594fa1b0c  TreatAsAtomicUnit=on
      mask Display: disp('CommFlt')
  CopyRight2 : Subsystem  Description=|  mask(Copyright Information){none=on}
      | Copyright info block.                                               
      |                                                                     
      | Place copyright information at the top of every subsystem in design.
      mask prompts: none "No parameters"
      mask help: Place copyright information at the top of every subsystem in design.
      mask Display:
      | NxtrConf = 'Nexteer Confidential';
      | 
      | sys = bdroot; %handle for the current model ("system")
      | first = get_param(sys,'Created');
      | first = first(end-3:end);  %year is last four digits
      | 
      | last = get_param(sys,'LastModifiedDate');
      | if isempty(last)
      |     last = datestr(now,'yyyy');
      | else
      |     last = last(end-3:end);
      | end
      | 
      | if strcmp(first,last)
      |     fprintf('%s -- Copyright %s Nexteer',NxtrConf,first)
      | else
      |     fprintf('%s -- %s%s- %s Nexteer',NxtrConf,char(169),first,last)
      | end
  If : If  IfExpression=u1 == 0
  Merge : Merge
  Merge1 : Merge
  Merge2 : Merge
  TestPass : Subsystem  RequirementInfo={'doors' '00006115' '20' 'false' 'DOORS Surrogate Item' '' ; 'linktype_rmi_doors' '0000c47c (/ESG Group/FDD Module Requirements/EA4 Specific/CM660A_HwTq1Meas)' '#CM660A_49' 'true' 'REQ: CM660A_49' '' } %GIDa_eb2d61f5_a171_4ae7_8550_49e90430938b  TreatAsAtomicUnit=on
      mask Display: disp('TESTPASS')
  Out1 : Outport
  wires:
  HwTq1FCCN/1 -> If/1
  If/1 -> TestPass/Action
  If/2 -> CommFlt/Action
  Merge/1 -> Bus Creator/2  "TestOk"
  Merge1/1 -> Bus Creator/3  "ParamByte"
  Merge2/1 -> Bus Creator/1  "RawHwTq"
  TestPass/1(Out1) -> Bus Selector/1
  CommFlt/1(Out2) -> Bus Selector1/1
  Bus Selector1/1 -> Merge2/1  "<RawHwTq>"
  Bus Selector/1 -> Merge2/2  "<RawHwTq>"
  Bus Selector1/2 -> Merge/1  "<TestOk>"
  Bus Selector1/3 -> Merge1/1  "<ParamByte>"
  Bus Selector/2 -> Merge/2  "<TestOk>"
  Bus Selector/3 -> Merge1/2  "<ParamByte>"
  Bus Creator/1 -> Out1/1
  HwTq1Data/1 -> TestPass/1(HwTq1Data)
